simulink model "SDRPart1"  (R2023a)
settings: Solver=FixedStepAuto  StartTime=0.0  StopTime=0.001  FixedStep=1/(80e6)  RelTol=1e-3
libraries: dspxfrm3 x1, dspsigops x1, simulink x1, commrandsrc3 x1
settings Model: Creator=User  LastModifiedBy=User

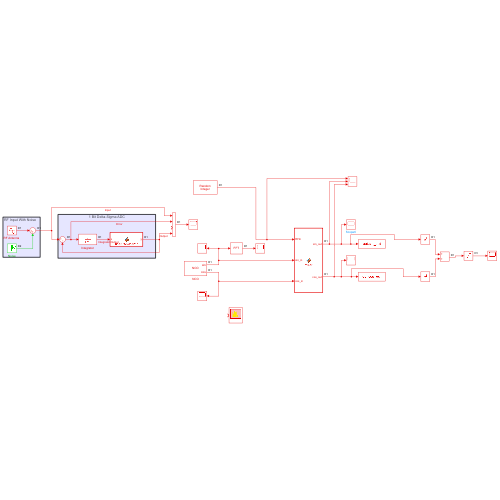
[thumbnail: Simulink's stored preview of the top-level diagram]
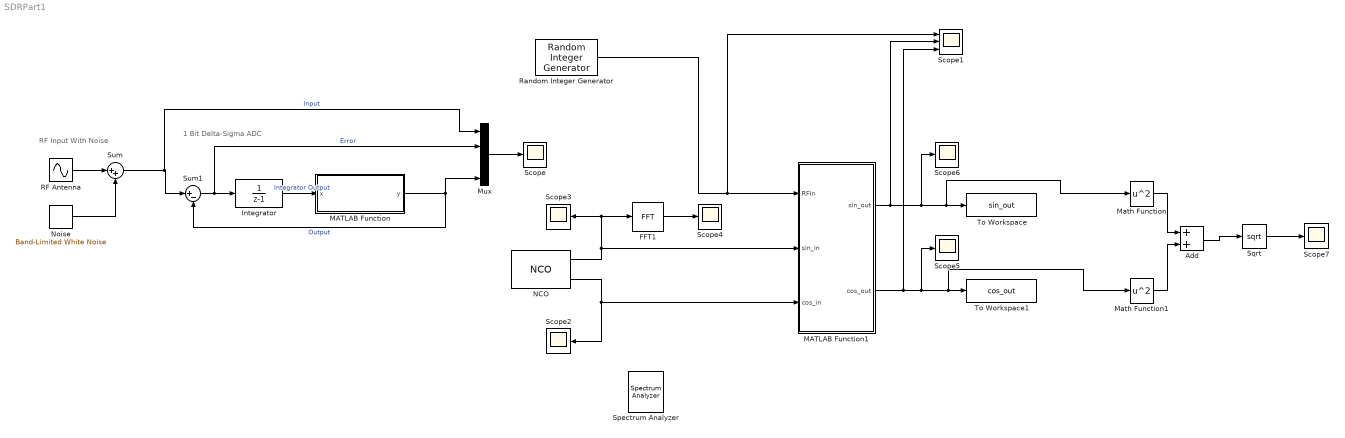
== system SDRPart1 ==
  note: RF Input With Noise
  note: 1 Bit Delta-Sigma ADC
  Add : Sum
  FFT1 : dspxfrm3/FFT  FFTImplementation=Auto  CompMethod=Table lookup  TableOpt=NEW  TableOptActive=Speed  BitRevOrder=off  Normalize=off  InheritFFTLength=on  FFTLength=64  WrapInput=on  roundingMode=Floor  overflowMode=off  firstCoeffDataTypeStr=Inherit: Same word length as input  firstCoeffLastDataTypeStr=Inherit: Same word length as input  outputMin=[]  outputMax=[]
  Integrator : DiscreteTransferFcn  Denominator=[1 -1]
  MATLAB Function : MATLAB Function  TreatAsAtomicUnit=on
  MATLAB Function1 : MATLAB Function  TreatAsAtomicUnit=on
  Math Function : Math  Operator=square
  Math Function1 : Math  Operator=square
  Mux : Mux
  NCO : dspsigops/NCO  AccIncSrc=Specify via dialog  AccInc=1530e3*2^64/(80e6)  PhaseOffsetSrc=Specify via dialog  PhaseOffset=0  AccumWL=64  HasDither=off  DitherWL=4  PNgeneratorLength=19  HasPhaseQuantizer=on  TableDepth=8  HasOutputPhaseError=off  Formula=Sine and cosine  DataType=Binary point scaling  OutputWL=16  OutputFL=5  CompMethod=Table lookup (no interpolation)  SampleTime=1/(80e6)  SamplesPerFrame=1  OutputFrames=off
      settings: LibrarySourceBlock=dspsrcs4/NCO
  Noise : simulink/Sources/Band-Limited White Noise  Cov=[0.001]  Ts=0.1  seed=[23341]
  "RF Antenna " : Sin  Frequency=2*pi*1530e3  SampleTime=1/(80e6)
  Random Integer Generator : commrandsrc3/Random Integer Generator  SetSize=2  SeedSource=Auto  Seed=0  SampleTime=1/80e6  SamplesPerFrame=1  OutputDataType=double  SimulateUsing=Interpreted execution
  Scope{,2..7} (7 alike) : Scope
  Scope1 : Scope  NumInputPorts=3
  Spectrum Analyzer : SpectrumAnalyzer  WindowPosition=[1.000000,41.000000,1920.000000,1017.000000,]  ScopeFrameLocation=window  SpectrumType=RMS  SampleRateSource=Property  SampleRate=80000000  StartFrequency=20  StopFrequency=20e3  SpectrumUnits=Vrms  YLimits=[-106.64125475,2.97669937]  ColorLimits=[-20 80]  ExpandToolstrip=on  SelectedToolstripTab=spectrumAnalyzerToolstrip.spectrumTab  DefaultConfigurationName=spbscopes.SpectrumAnalyzerBlockCfg  IsFrequencyInputMode=0  FrequencyVectorPort=0  FrequencyVectorFromPort=0  FrequencyInputRBWPort=0  FrequencyInputRBWFromPort=0
  Sqrt : Sqrt
  Sum : Sum  Inputs=|++
  Sum1 : Sum  Inputs=|+-
  To Workspace : ToWorkspace  VariableName=sin_out  SaveFormat=Structure With Time  SampleTime=-1
  To Workspace1 : ToWorkspace  VariableName=cos_out  SaveFormat=Structure With Time  SampleTime=-1
  wires:
  Noise/1 -> Sum/2
  "RF Antenna "/1 -> Sum/1
  Integrator/1 -> MATLAB Function/1(x)  "Integrator Output"
  Sum1/1 -> Mux/2, Integrator/1  "Error"
  Sum/1 -> Mux/1, Sum1/1  "Input"
  MATLAB Function/1(y) -> Mux/4, Sum1/2  "Output"
  Mux/1 -> Scope/1
  NCO/2 -> Scope2/1, MATLAB Function1/3(cos_in)
  MATLAB Function1/1(sin_out) -> Scope1/2, Scope6/1, Math Function/1, To Workspace/1
  MATLAB Function1/2(cos_out) -> Scope1/3, Scope5/1, Math Function1/1, To Workspace1/1
  FFT1/1 -> Scope4/1
  NCO/1 -> MATLAB Function1/2(sin_in), Scope3/1, FFT1/1
  Sqrt/1 -> Scope7/1
  Add/1 -> Sqrt/1
  Math Function/1 -> Add/1
  Math Function1/1 -> Add/2
  Random Integer Generator/1 -> Scope1/1, MATLAB Function1/1(RFIn)

== matlab function SDRPart1/MATLAB Function1 ==
  data: RFIn input; sin_out output; sin_in input; cos_in input; cos_out output
function [sin_out, cos_out] = mixer(RFIn, sin_in, cos_in)
    % Check the value of RFIn to determine if the sin and cos values
    % should be negated or not.
    if RFIn == 1
        sin_out = sin_in;
        cos_out = cos_in;
    else
        sin_out = -sin_in;
        cos_out = -cos_in;
    end
end

== matlab function SDRPart1/MATLAB Function ==
  data: x input; y output
function y = oneBitQuantizer(x)
% Simple 1-bit quantizer function
if x >= 0
    y = 1;
else
    y = -1; % y=0?
end
